simulink model "Modello_Irb1300"  (R2024a)
settings: Solver=VariableStepAuto  StartTime=0.0  StopTime=37  RelTol=1e-3
undefined symbols (not defined in the file or in its folder): DiscIntNeverNeededParam
libraries: vrlib x3, simulink x1
(part 2 of 2)

== matlab function Modello_Irb1300/MATLAB Function3 ==
  data: collison_R input; R_position input; O_d input; mode input; o output; pos output
function [o,pos] = posa_spina(collison_R,R_position,O_d,mode)
     
     
     
     psi = O_d(3); % Rotazione attorno all'asse Z dell'end effector (Asse che punta verso il pezzo da agganciare)

     pos = [0.60; 0.7; 0.4];
     o = [0 0 0 0];

     
     
     % Viene utilizzata la matrice di rotazione R_robot_to_scene per
     % traformare la posizione del dell'end effector riferita alla terna
     % del robot R_position, in posizione dell'end effector riferita alla
     % scena
     R_robot_to_scene = [1,   0,   0;     
                         0,   0,   1;     
                         0,  -1,   0];
     
    robot_pos = R_robot_to_scene * R_position;
    
    %utilizziamo la variabile mode per individuare quale tipo Task abbiamo
    %simulando in questo modo possiamo impostare nel modo giusto la
    %posizione della spina 
    
    % Inizializzazione della variabile sgancio_spina di tipo persistente,
    % in questo modo è possibile tenere conto dello stato della variabile
    % in ogni istante mantenedo lo stato anche dopo il controllo

    persistent sgancio_spina;
    
     if isempty(sgancio_spina)
       sgancio_spina = 0;
    end
 

     %pos = R_robot_to_scene * R_position;
    if (mode == 0)
        %pos = [0.60; 0.7; 0.4];  % posizione costante (x, z, y) [0.39 0.45 -0.31];
        if (collison_R == 1)
            pos = robot_pos;
        % display(pos);
            if (psi == -pi/2)
                o = [1 0 0 -1.5708];
            end
             % display('x');
             % display(robot_pos(1));
             % display('y');
             % display(robot_pos(2));
             % display('z');
             % display(robot_pos(3));  
        end
        if((abs(robot_pos(1) - 0.55) < 0.02) && (abs(robot_pos(2) - 0.57) < 0.02) && (abs(robot_pos(3) - 0.14) < 0.02))
            sgancio_spina = 1;
        end
        if(sgancio_spina == 1)
             pos = [0.55; 0.57; 0.14];
             o = [1 0 0 -1.5708];
        end

    elseif(mode == 1)

        pos = [0.55; 0.57; 0.14];
        o = [1 0 0 -1.5708];
        if (collison_R == 1)
            pos = robot_pos;
            if (psi == -pi/2)
                o = [1 0 0 -1.5708];
            elseif (psi == 0)
                 o = [1 0 0 0];
            end
            
        end

        if((abs(robot_pos(1) - 0.55) < 0.005) && (abs(robot_pos(2) - 0.70) < 0.005) && (abs(robot_pos(3) - 0.45) < 0.005))
            sgancio_spina = 1;
        end

        if(sgancio_spina == 1)
             pos = [0.55; 0.70; 0.45];
             o = [1 0 0 0];
        end
    end
end

      % if (collison_R == 1)
    %     pos = R_robot_to_scene * R_position;
    %    display(pos);
    % end
    % if (collison_R == 1 && psi == -pi/2)
    %     o = [1 0 0 -1.5708];
    %    display(o);
    % end

== matlab function Modello_Irb1300/MATLAB Function4 ==
  data: i1 input; y output; i2 input
function y  = collision_detection(i1, i2)
   % Trasformazione dal frame della scena al frame del robot
   R_scene_to_robot = [1,  0,  0;     % x_s -> x_r
                       0,  0, -1;     % z_s -> -y_r
                       0, 1,   0];    % y_s -> z_r

   % Applicazione della trasformazione a i1
   i1_robot = R_scene_to_robot * i1;

   % Coordinate di i1 nel frame del robot

   xi1 = i1_robot(1); % Asse X del robot
   yi1 = i1_robot(2); % Asse Y del robot
   zi1 = i1_robot(3); % Asse Z del robot

   % Coordinate di i2 nel frame del robot
   xi2 = i2(1,1);
   yi2 = i2(2,1);
   zi2 = i2(3,1);

   % Inizializzazione del risultato
   y = 0;

   % Controllo collisione
   if ((abs(xi1 - xi2) < 0.02) && (abs(yi1 - yi2) < 0.02) && (abs(zi1 - zi2) < 0.02))
       y = 1;
   end
end

== matlab function Modello_Irb1300/MATLAB Function5 ==
  data: Vp input; V output; Omega input
function V = fcn(Vp,Omega)
% Questa funzione a partire dalle velocità delle Velocità Vp e le
% orientazioni creo il vettore V [6x1]
V = [Vp;Omega];

== matlab function Modello_Irb1300/MATLAB Function6 ==
  data: O_d input; R_error output; R_a input
function R_error = Orientation(O_d,R_a)
% R_a, è la matrice di rotazione ottenuta dalla posa in retroazione 

%R_iniziale, questa matrice è la matrice iniziale (orientazione assoluta) 
%che permette di riferire gli angoli di eulero alla orientazione relativa dell'end effector

R_iniziale = [
    0.0000    0.0000    1.0000 ;
    1.0000         0    0.0000 ;
         0    1.0000    0.0000 ];

% Angoli pi di Eulero in radianti
theta = O_d(1);          % Rotazione attorno all'asse x 
  phi = O_d(2);          % Rotazione attorno all'asse y 
  psi = O_d(3) + pi/2 ;  % Rotazione attorno all'asse z (per corretta posizione a riposo)

% Matrici di rotazione elementari
R_x = [
      1, 0, 0;
      0, cos(theta), -sin(theta);
      0, sin(theta), cos(theta)
];

R_y = [
    cos(phi), 0, sin(phi);
    0, 1, 0;
    -sin(phi), 0, cos(phi)
];

R_z = [
    cos(psi), -sin(psi), 0;
    sin(psi), cos(psi), 0;
    0, 0, 1
];

% Matrice di rotazione totale
% R_d_rel consiste nella matrice di Rotazione Desiderate relativa all'endeffector
R_d_rel = R_z * R_y * R_x;  % Ordine: ZYX (dipende dalla convenzione scelta)

%R_d_ass consiste nella matrice di rotazione desiderata assoluta espressa
%rispetto la terna di base del robot 
R_d_ass = R_iniziale * R_d_rel;

% Calcolo del'errore angolare R_error
% Prodotto della matrice di rotazione desderata per la trasposta
% della matrice di Rotazione attuale 
R_error = R_d_ass * R_a';

end

% function omega_e = calcOmegaError(R_d, R_a)
%     % Calcola la matrice di errore
%     R_error = R_d * R_a';
% 
%     % Calcola theta
%     theta = acos((trace(R_error) - 1) / 2);
% 
%     % Calcola matrice antisimmetrica u_hat
%     if abs(sin(theta)) > 1e-6  % Evita divisioni per zero
%         u_hat = (R_error - R_error') / (2 * sin(theta));
%     else
%         u_hat = zeros(3);  % Caso limite (errore molto piccolo)
%     end
% 
%     % Estrai omega_e usando vex
%     omega_e = [u_hat(3, 2); u_hat(1, 3); u_hat(2, 1)];
% end
% 
% 






% % Angoli di Eulero in radianti
% theta = pi/6;  % Rotazione attorno all'asse x (30°)
% phi = pi/4;    % Rotazione attorno all'asse y (45°)
% psi = pi/3;    % Rotazione attorno all'asse z (60°)
% 
% % Matrici di rotazione elementari
% R_x = [
%     1, 0, 0;
%     0, cos(theta), -sin(theta);
%     0, sin(theta), cos(theta)
% ];
% R_y = [
%     cos(phi), 0, sin(phi);
%     0, 1, 0;
%     -sin(phi), 0, cos(phi)
% ];
% R_z = [
%     cos(psi), -sin(psi), 0;
%     sin(psi), cos(psi), 0;
%     0, 0, 1
% ];
% 
% % Matrice di rotazione totale
% R_d = R_z * R_y * R_x;  % Ordine: ZYX (dipende dalla convenzione scelta)

% % Inizializzo la matrice che definisce l'orientazione desidarata 
% % In questo esempio, R_d è una matrice di rotazione che rappresenta una rotazione 
% % di 30° rispetto all'asse Z.
% R_d = [0.866, -0.5, 0;
%        0.5,  0.866, 0;
%          0,      0, 1];

== matlab function Modello_Irb1300/MATLAB Function7 ==
  data: R_error input; omega output
% function omega = calcAngularVelocity(R_error)
%     omega = 0.5 * [
%         R_error(3,2) - R_error(2,3);
%         R_error(1,3) - R_error(3,1);
%         R_error(2,1) - R_error(1,2)
%     ];
% end

 function omega = calcOmegaError(R_error)
    % Calcola la matrice di errore

    % Calcola theta
    theta = acos((trace(R_error) - 1) / 2);

    % Calcola matrice antisimmetrica u_hat
    if abs(theta) < 1e-6  % Evita divisioni per zero
        omega = [0;0;0];
    else
        skew_matrix = (R_error - R_error')/(2*sin(theta));  % Caso limite (errore molto piccolo)
        omega = [skew_matrix(3,2);skew_matrix(1,3);skew_matrix(2,1)];
    end

    % Estrai omega_e usando vex
    omega = theta * omega;
end
